simulink model "sp"  (R2018a)
settings: Solver=VariableStepAuto  StartTime=0.0  StopTime=sim_time  RelTol=1e-9
values from neighbouring files (symbols this model uses):
  ICs = [y_IC deg2rad(0)]    [setpoint_block.m]
  L = 1.524    [setpoint_block.m]
  V = 4.5    [setpoint_block.m]
  vehicleIC = [track_vector(1,1)-y_IC*sin(ICs(2)) track_vector(1,2)+y_IC*cos(ICs(2))]    [setpoint_block.m]
undefined symbols (not defined in the file or in its folder): K
settings Model: Creator=journeyman  LastModifiedBy=journeyman

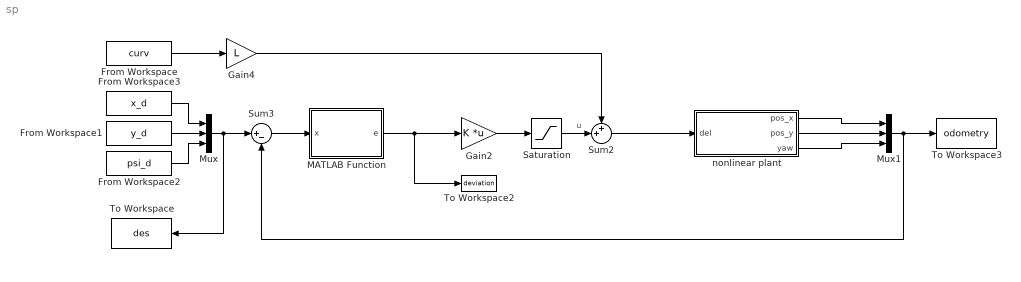
== system sp ==
  From Workspace : FromWorkspace  VariableName=curv  SampleTime=0
  From Workspace1 : FromWorkspace  VariableName=y_d  SampleTime=0
  From Workspace2 : FromWorkspace  VariableName=psi_d  SampleTime=0
  From Workspace3 : FromWorkspace  VariableName=x_d  SampleTime=0
  Gain2 : Gain  Gain=K  Multiplication=Matrix(K*u)
  Gain4 : Gain  Gain=L
  MATLAB Function : MATLAB Function  TreatAsAtomicUnit=on
  Mux : Mux  Inputs=3
  Mux1 : Mux  Inputs=3
  Saturation : Saturate  UpperLimit=deg2rad(30)  LowerLimit=deg2rad(-30)
  Sum2 : Sum  Inputs=++|
  Sum3 : Sum  Inputs=|+-
  To Workspace : ToWorkspace  VariableName=des  SampleTime=-1
  To Workspace2 : ToWorkspace  VariableName=deviation  SampleTime=-1
  To Workspace3 : ToWorkspace  VariableName=odometry  SampleTime=-1
  nonlinear plant : Subsystem
  wires:
  nonlinear plant/2(pos_y) -> Mux1/2
  From Workspace/1 -> Gain4/1
  Sum2/1 -> nonlinear plant/1(del)
  Mux/1 -> To Workspace/1, Sum3/1
  Gain2/1 -> Saturation/1
  Sum3/1 -> MATLAB Function/1(x)
  Saturation/1 -> Sum2/2  "u"
  From Workspace2/1 -> Mux/3
  From Workspace1/1 -> Mux/2
  From Workspace3/1 -> Mux/1
  Mux1/1 -> Sum3/2, To Workspace3/1
  nonlinear plant/1(pos_x) -> Mux1/1
  nonlinear plant/3(yaw) -> Mux1/3
  MATLAB Function/1(e) -> Gain2/1, To Workspace2/1
  Gain4/1 -> Sum2/1

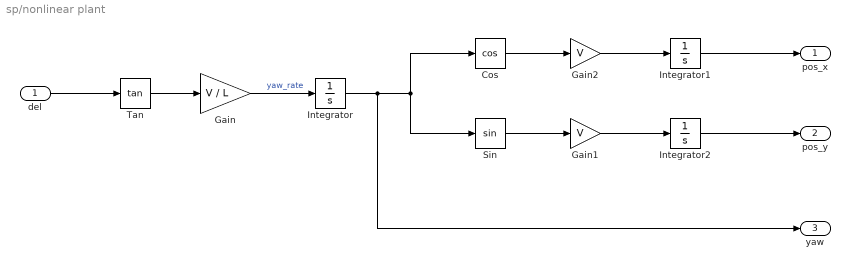
== system sp/nonlinear plant ==
  del : Inport
  Cos : Trigonometry  Operator=cos
  Gain : Gain  Gain=V / L
  Gain1 : Gain  Gain=V
  Gain2 : Gain  Gain=V
  Integrator : Integrator  InitialCondition=ICs(2)
  Integrator1 : Integrator  InitialCondition=vehicleIC(1)
  Integrator2 : Integrator  InitialCondition=vehicleIC(2)
  Sin : Trigonometry
  Tan : Trigonometry  Operator=tan
  pos_x : Outport
  pos_y : Outport  Port=2
  yaw : Outport  Port=3
  wires:
  del/1 -> Tan/1
  Tan/1 -> Gain/1
  Gain/1 -> Integrator/1  "yaw_rate"
  Integrator/1 -> yaw/1, Sin/1, Cos/1
  Sin/1 -> Gain1/1
  Cos/1 -> Gain2/1
  Gain2/1 -> Integrator1/1
  Gain1/1 -> Integrator2/1
  Integrator2/1 -> pos_y/1
  Integrator1/1 -> pos_x/1

== matlab function sp/MATLAB Function ==
  data: x input; e output
function e = DCM(x)

DCM = @(ang) [cos(ang) sin(ang) 0;
             -sin(ang) cos(ang) 0;
             0            0     1];
E = DCM(x(3))*x;
e = E(2:3, 1);
